simulink model "simulink_q8"  (R2020a)
settings: Solver=VariableStepAuto  StartTime=0.0  StopTime=50  RelTol=1e-3
settings Model: Creator=debora  LastModifiedBy=debora

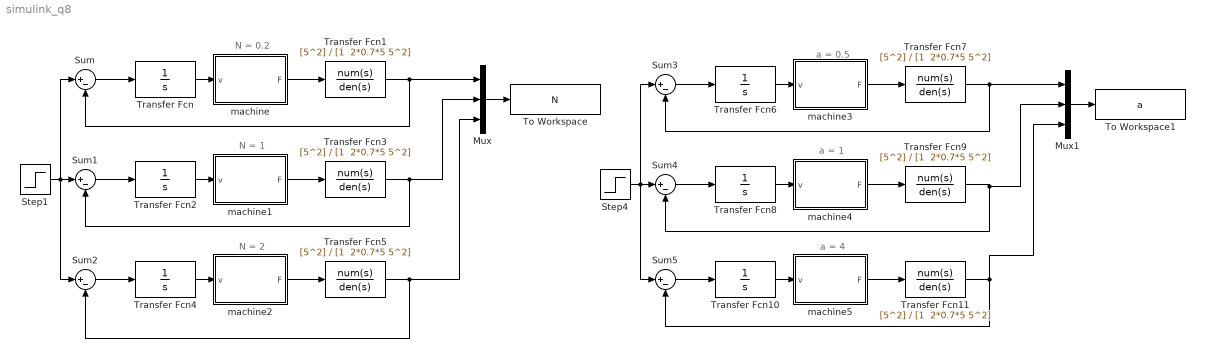
== system simulink_q8 ==
  note: N = 2
  note: N = 1
  note: N = 0.2
  note: a = 0.5
  note: a = 1
  note: a = 4
  Mux : Mux  Inputs=3
  Mux1 : Mux  Inputs=3
  Step1 : Step  Time=0  SampleTime=0
  Step4 : Step  Time=0  SampleTime=0
  Sum{,1..5} (6 alike) : Sum  Inputs=|+-
  To Workspace : ToWorkspace  VariableName=N  SaveFormat=Timeseries  SampleTime=-1
  To Workspace1 : ToWorkspace  VariableName=a  SaveFormat=Timeseries  SampleTime=-1
  Transfer Fcn{,2,4,6,8,10} (6 alike) : TransferFcn  Denominator=[1 0]
  Transfer Fcn{1,3,5,7,9,11} (6 alike) : TransferFcn  Numerator=[5^2]  Denominator="[1  2*0.7*5 5^2]"
  machine : MATLAB Function  TreatAsAtomicUnit=on
  machine1 : MATLAB Function  TreatAsAtomicUnit=on
  machine2 : MATLAB Function  TreatAsAtomicUnit=on
  machine3 : MATLAB Function  TreatAsAtomicUnit=on
  machine4 : MATLAB Function  TreatAsAtomicUnit=on
  machine5 : MATLAB Function  TreatAsAtomicUnit=on
  wires:
  Step1/1 -> Sum/1, Sum1/1, Sum2/1
  Sum/1 -> Transfer Fcn/1
  Transfer Fcn/1 -> machine/1(v)
  machine/1(F) -> Transfer Fcn1/1
  Transfer Fcn1/1 -> Mux/1, Sum/2
  Transfer Fcn3/1 -> Mux/2, Sum1/2
  Sum1/1 -> Transfer Fcn2/1
  Transfer Fcn2/1 -> machine1/1(v)
  machine1/1(F) -> Transfer Fcn3/1
  Transfer Fcn5/1 -> Mux/3, Sum2/2
  Sum2/1 -> Transfer Fcn4/1
  Transfer Fcn4/1 -> machine2/1(v)
  machine2/1(F) -> Transfer Fcn5/1
  Transfer Fcn7/1 -> Mux1/1, Sum3/2
  Step4/1 -> Sum3/1, Sum5/1, Sum4/1
  Transfer Fcn6/1 -> machine3/1(v)
  Sum3/1 -> Transfer Fcn6/1
  machine3/1(F) -> Transfer Fcn7/1
  Sum4/1 -> Transfer Fcn8/1
  machine4/1(F) -> Transfer Fcn9/1
  Transfer Fcn8/1 -> machine4/1(v)
  Transfer Fcn9/1 -> Mux1/2, Sum4/2
  machine5/1(F) -> Transfer Fcn11/1
  Sum5/1 -> Transfer Fcn10/1
  Transfer Fcn11/1 -> Mux1/3, Sum5/2
  Transfer Fcn10/1 -> machine5/1(v)
  Mux/1 -> To Workspace/1
  Mux1/1 -> To Workspace1/1

== matlab function simulink_q8/machine ==
  data: v input; F output
function F = fcn(v)
    alpha = 0.7;
    k = 1;
    a = 1;
    N = 0.2;
    F = k*a*(v/N)^alpha;
end

== matlab function simulink_q8/machine2 ==
  data: v input; F output
function F = fcn(v)
    alpha = 0.7;
    k = 1;
    a = 1;
    N = 2;
    F = k*a*(v/N)^alpha;
end

== matlab function simulink_q8/machine3 ==
  data: v input; F output
function F = fcn(v)
    alpha = 0.7;
    k = 1;
    a = 0.5;
    N = 1;
    F = k*a*(v/N)^alpha;
end

== matlab function simulink_q8/machine4 ==
  data: v input; F output
function F = fcn(v)
    alpha = 0.7;
    k = 1;
    a = 1;
    N = 1;
    F = k*a*(v/N)^alpha;
end

== matlab function simulink_q8/machine5 ==
  data: v input; F output
function F = fcn(v)
    alpha = 0.7;
    k = 1;
    a = 4;
    N = 1;
    F = k*a*(v/N)^alpha;
end

== matlab function simulink_q8/machine1 ==
  data: v input; F output
function F = fcn(v)
    alpha = 0.7;
    k = 1;
    a = 1;
    N = 1;
    F = k*a*(v/N)^alpha;
end
